simulink model "exer_2_2_4"  (R2014b)
settings: Solver=ode45  StartTime=0.0  StopTime=10.0  RelTol=1e-3
libraries: dspsnks4 x1
settings Model: Creator=Charlie  LastModifiedBy=Charlie

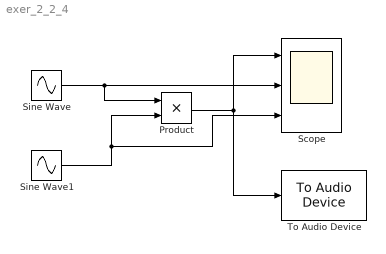
== system exer_2_2_4 ==
  Product : Product
  Scope : Scope  NumInputPorts=3
      settings: YMin=-5~-5~-5  YMax=5~5~5
  Sine Wave : Sin  Frequency=31.25  SampleTime=1/48000
  Sine Wave1 : Sin  Frequency=500  SampleTime=1/48000
  To Audio Device : dspsnks4/To Audio Device  deviceName=Default  inheritSampleRate=on  sampleRate=44100  deviceDatatype=Determine from input data type  autoBufferSize=on  bufferSize=4096  queueDuration=1.0  defaultOutputChannelMapping=on  outputChannelMapping=1:2  outputNumUnderrunSamples=off
  wires:
  Sine Wave/1 -> Scope/2, Product/1
  Sine Wave1/1 -> Scope/3, Product/2
  Product/1 -> To Audio Device/1, Scope/1
